simulink model "DictionaryExample"  (R2025b)
settings: Solver=VariableStepAuto  StartTime=0.0  StopTime=10.0  RelTol=1e-3
model workspace (MAT data in the model file):
  DataInterface = Simulink.Bus
  DataInterface.Alignment = -1
  DataInterface.PreserveElementDimensions = 0
  DataInterface.Elements_internal = Simulink.BusElement
  DataInterface.Elements_internal.DimensionsMode = 'Fixed'
  DataInterface.Elements_internal.SamplingMode = 'Sample based'
  DataInterface.Elements_internal.SampleTime = -1
  DataInterface.Elements_internal.Name = 'Element1'
  DataInterface.Elements_internal.DataType_internal = 'double'
  DataInterface.Elements_internal.Complexity = 'real'
  DataInterface.Elements_internal.Dimensions = 1
  DataInterface.DataScope = 'Auto'
  DataInterface1 = Simulink.Bus
  DataInterface1.Alignment = -1
  DataInterface1.PreserveElementDimensions = 0
  DataInterface1.Elements_internal = Simulink.BusElement
  DataInterface1.Elements_internal.DimensionsMode = 'Fixed'
  DataInterface1.Elements_internal.SamplingMode = 'Sample based'
  DataInterface1.Elements_internal.SampleTime = -1
  DataInterface1.Elements_internal.Name = 'Element2'
  DataInterface1.Elements_internal.DataType_internal = 'int64'
  DataInterface1.Elements_internal.Complexity = 'real'
  DataInterface1.Elements_internal.Dimensions = 1
  DataInterface1.DataScope = 'Auto'
settings Model: Creator=georg  LastModifiedBy=georg

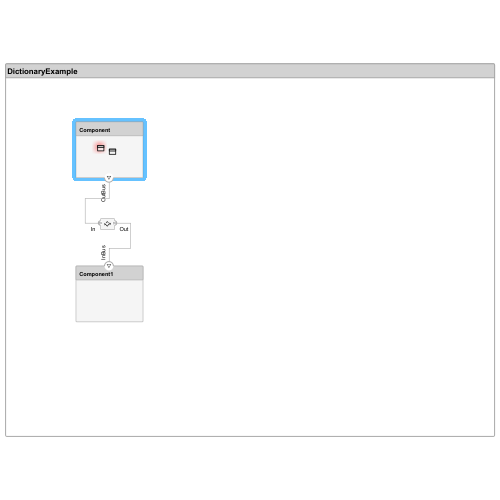
[thumbnail: Simulink's stored preview of the top-level diagram]
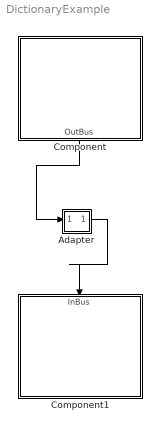
== system DictionaryExample ==
  Adapter : Subsystem
      settings: PortSchema="{\"entries\":[{\"content\":{\"margin\":10,\"minimumSpacing\":15,\"sides\":[{\"content\":{\"connectorIds\":[\"In1\"]},\"type\":\"ConnectorPlacement.EquallySpacedRectSide\",\"uuid\":\"8d645fa3-2e17-47d6-b57c-061bf9ca2ad7\"},{\"content\":{\"connectorIds\":[\"Out1\"],\"side\":\"RIGHT\"},\"type\":\"ConnectorPlacement.EquallySpacedRectSide\",\"uuid\":\"da1024a9-13df-487c-8b1b-4ef52eaa82ca\"},{\"content\":{\"side\":\"TOP\"},\"type\":\"ConnectorPlacement.EquallySpacedRectSide\",\"uuid\":\"4b7ed5f6-e467-4f05-b247-196e9d305cb8\"}]},\"type\":\"ConnectorPlacement.EquallySpacedConnector\",\"uuid\":\"d256ca4d-3894-42a0-b30b-ffcbc62b7626\"}],\"packageUris\":[\"http://schema.mathworks.com/mf0/Connector/R2020b\"],\"version\":\"1.0\"}"
  Component : Subsystem
      settings: PortSchema="{\"entries\":[{\"content\":{\"headerSize\":26,\"margin\":15,\"minimumSpacing\":25,\"sides\":[{\"content\":{},\"type\":\"ConnectorPlacement.EquallySpacedRectSide\",\"uuid\":\"8d645fa3-2e17-47d6-b57c-061bf9ca2ad7\"},{\"content\":{\"side\":\"RIGHT\"},\"type\":\"ConnectorPlacement.EquallySpacedRectSide\",\"uuid\":\"da1024a9-13df-487c-8b1b-4ef52eaa82ca\"},{\"content\":{\"side\":\"TOP\"},\"type\":\"ConnectorPlacement.EquallySpacedRectSide\",\"uuid\":\"4b7ed5f6-e467-4f05-b247-196e9d305cb8\"},{\"content\":{\"connectorIds\":[\"Out1\"],\"side\":\"BOTTOM\"},\"type\":\"ConnectorPlacement.EquallySpacedRectSide\",\"uuid\":\"f10afce5-09ba-4686-85c2-4bf98e57d5ba\"}]},\"type\":\"ConnectorPlacement.EquallySpacedConnector\",\"uuid\":\"d256ca4d-3894-42a0-b30b-ffcbc62b7626\"}],\"packageUris\":[\"http://schema.mathworks.com/mf0/Connector/R2020b\"],\"version\":\"1.0\"}"
  Component1 : Subsystem
      settings: PortSchema="{\"entries\":[{\"content\":{\"headerSize\":26,\"margin\":15,\"minimumSpacing\":25,\"sides\":[{\"content\":{},\"type\":\"ConnectorPlacement.EquallySpacedRectSide\",\"uuid\":\"8d645fa3-2e17-47d6-b57c-061bf9ca2ad7\"},{\"content\":{\"side\":\"RIGHT\"},\"type\":\"ConnectorPlacement.EquallySpacedRectSide\",\"uuid\":\"da1024a9-13df-487c-8b1b-4ef52eaa82ca\"},{\"content\":{\"connectorIds\":[\"In1\"],\"side\":\"TOP\"},\"type\":\"ConnectorPlacement.EquallySpacedRectSide\",\"uuid\":\"4b7ed5f6-e467-4f05-b247-196e9d305cb8\"}]},\"type\":\"ConnectorPlacement.EquallySpacedConnector\",\"uuid\":\"d256ca4d-3894-42a0-b30b-ffcbc62b7626\"}],\"packageUris\":[\"http://schema.mathworks.com/mf0/Connector/R2020b\"],\"version\":\"1.0\"}"
  wires:
  Adapter/1(Out) -> Component1/1(InBus)
  Component/1(OutBus) -> Adapter/1(In)

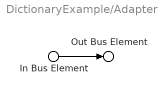
== system DictionaryExample/Adapter ==
  In Bus Element : Inport  PortName=In  Element=Element1
  Out Bus Element : Outport  PortName=Out  Element=Element2
  wires:
  In Bus Element/1 -> Out Bus Element/1

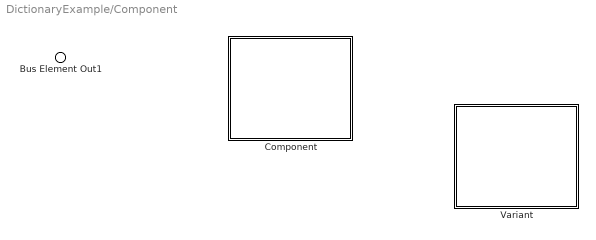
== system DictionaryExample/Component ==
  Component : ModelReference  SimulationMode=Normal
      settings: PortSchema="{\"entries\":[{\"content\":{\"headerSize\":38,\"margin\":15,\"minimumSpacing\":25,\"sides\":[{\"content\":{},\"type\":\"ConnectorPlacement.EquallySpacedRectSide\",\"uuid\":\"ff37e819-8e18-4faf-9e3b-d7311221fb5c\"},{\"content\":{\"side\":\"RIGHT\"},\"type\":\"ConnectorPlacement.EquallySpacedRectSide\",\"uuid\":\"72ac86a8-37e3-492d-b5cb-d8808905d6ab\"},{\"content\":{\"side\":\"TOP\"},\"type\":\"ConnectorPlacement.EquallySpacedRectSide\",\"uuid\":\"e669e504-7d16-4f43-b54e-584620db7182\"}]},\"type\":\"ConnectorPlacement.EquallySpacedConnector\",\"uuid\":\"8938ffdd-0d78-4165-bb91-be9f786776d7\"}],\"packageUris\":[\"http://schema.mathworks.com/mf0/Connector/R2020b\"],\"version\":\"1.0\"}"
  Variant : Subsystem  Variant=on  VariantControlMode=label  LabelModeActiveChoice=true
      settings: PortSchema="{\"entries\":[{\"content\":{\"headerSize\":38,\"margin\":15,\"minimumSpacing\":25,\"sides\":[{\"content\":{},\"type\":\"ConnectorPlacement.EquallySpacedRectSide\",\"uuid\":\"4982867e-7acf-4f3d-a21a-4fc903b10e0d\"},{\"content\":{\"side\":\"RIGHT\"},\"type\":\"ConnectorPlacement.EquallySpacedRectSide\",\"uuid\":\"22ff11be-278b-4bc0-87b8-a37262f0f0b5\"},{\"content\":{\"side\":\"TOP\"},\"type\":\"ConnectorPlacement.EquallySpacedRectSide\",\"uuid\":\"cd3f4465-7578-4ba1-bbc5-fd7b1ee57064\"}]},\"type\":\"ConnectorPlacement.EquallySpacedConnector\",\"uuid\":\"cff580b1-2a7b-487f-aa72-95d5c4f07942\"}],\"packageUris\":[\"http://schema.mathworks.com/mf0/Connector/R2020b\"],\"version\":\"1.0\"}"
  Bus Element Out1 : Outport  PortName=OutBus

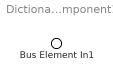
== system DictionaryExample/Component1 ==
  Bus Element In1 : Inport  PortName=InBus

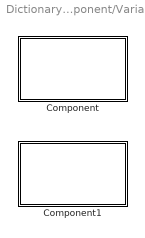
== system DictionaryExample/Component/Variant ==
  Component : Subsystem  VariantControl=true
      settings: PortSchema="{\"entries\":[{\"content\":{\"headerSize\":26,\"margin\":15,\"minimumSpacing\":25,\"sides\":[{\"content\":{},\"type\":\"ConnectorPlacement.EquallySpacedRectSide\",\"uuid\":\"f28b337a-df6f-4057-bcb4-4e6954610af1\"},{\"content\":{\"side\":\"RIGHT\"},\"type\":\"ConnectorPlacement.EquallySpacedRectSide\",\"uuid\":\"fd1c39fc-c976-4edc-9df3-bc75e22738e7\"},{\"content\":{\"side\":\"TOP\"},\"type\":\"ConnectorPlacement.EquallySpacedRectSide\",\"uuid\":\"574564af-2fdb-4991-a98a-ce01955867e8\"}]},\"type\":\"ConnectorPlacement.EquallySpacedConnector\",\"uuid\":\"b8588a05-b806-4451-99c3-aac5fd50c163\"}],\"packageUris\":[\"http://schema.mathworks.com/mf0/Connector/R2020b\"],\"version\":\"1.0\"}"
  Component1 : Subsystem  VariantControl=false
      settings: PortSchema="{\"entries\":[{\"content\":{\"headerSize\":26,\"margin\":15,\"minimumSpacing\":25,\"sides\":[{\"content\":{},\"type\":\"ConnectorPlacement.EquallySpacedRectSide\",\"uuid\":\"f28b337a-df6f-4057-bcb4-4e6954610af1\"},{\"content\":{\"side\":\"RIGHT\"},\"type\":\"ConnectorPlacement.EquallySpacedRectSide\",\"uuid\":\"fd1c39fc-c976-4edc-9df3-bc75e22738e7\"},{\"content\":{\"side\":\"TOP\"},\"type\":\"ConnectorPlacement.EquallySpacedRectSide\",\"uuid\":\"574564af-2fdb-4991-a98a-ce01955867e8\"}]},\"type\":\"ConnectorPlacement.EquallySpacedConnector\",\"uuid\":\"b8588a05-b806-4451-99c3-aac5fd50c163\"}],\"packageUris\":[\"http://schema.mathworks.com/mf0/Connector/R2020b\"],\"version\":\"1.0\"}"

== system DictionaryExample/Component/Variant/Component ==

== system DictionaryExample/Component/Variant/Component1 ==
